simulink model "NREL5MW_FBSWE_SLOW3DOF_IPC"  (R2021b)
settings: Solver=ode4  StartTime=0.0  StopTime=Parameter.Time.TMax  FixedStep=Parameter.Time.dt  RelTol=1e-3  EnableMultiTasking=on
values from neighbouring files (symbols this model uses):
  Parameter = NREL5MWDefaultParameter_FBSWE_IPC(Parameter)    [Exercise09_IndividualPitchControllerTest.m]
undefined symbols (not defined in the file or in its folder): x2_max, x2_min, x2_t0
libraries: simulink x4
(part 1 of 2)
settings Model: Creator=Phoenix_Shao  LastModifiedBy=david
settings SolverCC: AlgebraicLoopSolver=TrustRegion
settings DataIOCC: MaxDataPoints=1000000  SaveFormat=Array  DSMLogging=off  ReturnWorkspaceOutputs=off
settings OptimizationCC: ExpressionDepthLimit=2147483647  InitFltsAndDblsToZero=on  EfficientMapNaN2IntZero=off  LifeSpan=inf
settings DebuggingCC: SaveWithParameterizedLinksMsg=none  UnderspecifiedInitializationDetection=Classic  MergeDetectMultiDrivingBlocksExec=none  SignalResolutionControl=TryResolveAllWithWarning  SolverPrmCheckMsg=warning  MultiTaskDSMMsg=warning  MultiTaskCondExecSysMsg=none  FcnCallInpInsideContextMsg=warning  AllowSymbolicDim=off  StateNameClashWarn=warning  SFUnexpectedBacktrackingDiag=warning  SFNoUnconditionalDefaultTransitionDiag=warning  SFExecutionAtInitializationDiag=none  SFMachineParentedDataDiag=warning  ArithmeticOperatorsInVariantConditions=warning
settings HardwareCC: ProdBitPerPointer=32  ProdBitPerSizeT=32  ProdBitPerPtrDiffT=32  ProdLargestAtomicFloat=None  ProdIntDivRoundTo=Undefined  ProdEndianess=Unspecified  ProdWordSize=32  ProdHWDeviceType=32-bit Generic  TargetBitPerPointer=64  TargetBitPerSizeT=64  TargetBitPerPtrDiffT=64  TargetLongLongMode=on  TargetIntDivRoundTo=Zero  TargetEndianess=LittleEndian  TargetWordSize=64  TargetHWDeviceType=MATLAB Host  ProdEqTarget=off
settings ModelReferenceCC: PropagateSignalLabelsOutOfModel=off
settings SFSimCC: SimUseLocalCustomCode=off  SimParseCustomCode=off  CustomCodeUndefinedFunction=UseInterfaceOnly
settings RTWCC: SystemTargetFile=accel.tlc  TemplateMakefile=accel_default_tmf  RTWVerbose=off  RTWUseLocalCustomCode=off
settings CodeAppCC: MaxIdLength=128  StateflowObjectComments=on
settings STFCustomTargetCC: MATLABClassNameForMDSCustomization=Simulink.SoftwareTarget.TargetSpecificTriggerConfigurationBase  SystemTargetFile=accel.tlc
settings ConfigComp: CovMetricSettings=dw  CovSaveCumulativeToWorkspaceVar=on  CovSaveSingleToWorkspaceVar=on  CovExternalEMLEnable=off

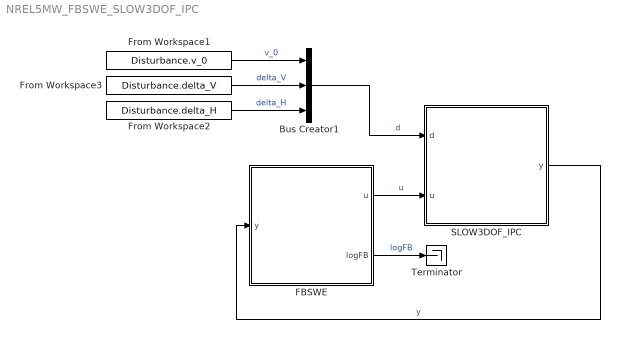
== system NREL5MW_FBSWE_SLOW3DOF_IPC ==
  Bus Creator1 : BusCreator  Inputs=3
  FBSWE : Subsystem
  From Workspace1 : FromWorkspace  VariableName=Disturbance.v_0
  From Workspace2 : FromWorkspace  VariableName=Disturbance.delta_H
  From Workspace3 : FromWorkspace  VariableName=Disturbance.delta_V
  SLOW3DOF_IPC : Subsystem
  Terminator : Terminator
  wires:
  SLOW3DOF_IPC/1(y) -> FBSWE/1(y)  "y"
  FBSWE/2(logFB) -> Terminator/1  "logFB"
  From Workspace1/1 -> Bus Creator1/1  "v_0"
  From Workspace3/1 -> Bus Creator1/2  "delta_V"
  From Workspace2/1 -> Bus Creator1/3  "delta_H"
  FBSWE/1(u) -> SLOW3DOF_IPC/2(u)  "u"
  Bus Creator1/1 -> SLOW3DOF_IPC/1(d)  "d"

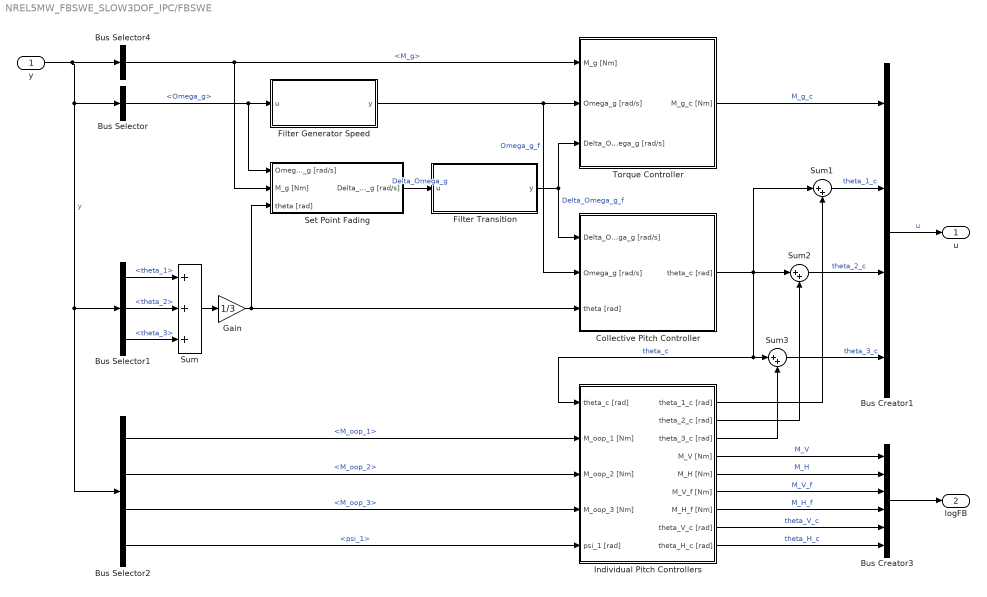
== system NREL5MW_FBSWE_SLOW3DOF_IPC/FBSWE ==
  y : Inport
  Bus Creator1 : BusCreator  Inputs=4
  Bus Creator3 : BusCreator  Inputs=6
  Bus Selector : BusSelector  OutputSignals=Omega_g
  Bus Selector1 : BusSelector  OutputSignals=theta_1,theta_2,theta_3
  Bus Selector2 : BusSelector  OutputSignals=M_oop_1,M_oop_2,M_oop_3,psi_1
  Bus Selector4 : BusSelector  OutputSignals=M_g
  Collective Pitch Controller : Subsystem
  Filter Generator Speed : Subsystem
  Filter Transition : Subsystem
  Gain : Gain  Gain=1/3
  Individual Pitch Controllers : Subsystem
  Set Point Fading : Subsystem
  Sum : Sum  Inputs=+++
  Sum1 : Sum  Inputs=|++
  Sum2 : Sum  Inputs=|++
  Sum3 : Sum  Inputs=|++
  Torque Controller : Subsystem
  u : Outport  VectorParamsAs1DForOutWhenUnconnected=off
  logFB : Outport  Port=2  VectorParamsAs1DForOutWhenUnconnected=off
  wires:
  Bus Selector/1 -> Set Point Fading/1(Omega_g [rad/s]), Filter Generator Speed/1(u)  "<Omega_g>"
  y/1 -> Bus Selector/1, Bus Selector2/1, Bus Selector1/1, Bus Selector4/1  "y"
  Torque Controller/1(M_g_c [Nm]) -> Bus Creator1/1  "M_g_c"
  Bus Creator1/1 -> u/1  "u"
  Filter Generator Speed/1(y) -> Collective Pitch Controller/2(Omega_g [rad/s]), Torque Controller/2(Omega_g [rad/s])  "Omega_g_f"
  Bus Selector4/1 -> Set Point Fading/2(M_g [Nm]), Torque Controller/1(M_g [Nm])  "<M_g>"
  Set Point Fading/1(Delta_Omega_g [rad/s]) -> Filter Transition/1(u)  "Delta_Omega_g"
  Filter Transition/1(y) -> Collective Pitch Controller/1(Delta_Omega_g [rad/s]), Torque Controller/3(Delta_Omega_g [rad/s])  "Delta_Omega_g_f"
  Bus Selector1/1 -> Sum/1  "<theta_1>"
  Bus Selector1/2 -> Sum/2  "<theta_2>"
  Bus Selector1/3 -> Sum/3  "<theta_3>"
  Sum/1 -> Gain/1
  Gain/1 -> Set Point Fading/3(theta [rad]), Collective Pitch Controller/3(theta [rad])
  Sum1/1 -> Bus Creator1/2  "theta_1_c"
  Sum2/1 -> Bus Creator1/3  "theta_2_c"
  Sum3/1 -> Bus Creator1/4  "theta_3_c"
  Collective Pitch Controller/1(theta_c [rad]) -> Sum1/1, Individual Pitch Controllers/1(theta_c [rad]), Sum3/1, Sum2/1  "theta_c"
  Bus Selector2/1 -> Individual Pitch Controllers/2(M_oop_1 [Nm])  "<M_oop_1>"
  Bus Selector2/2 -> Individual Pitch Controllers/3(M_oop_2 [Nm])  "<M_oop_2>"
  Bus Selector2/3 -> Individual Pitch Controllers/4(M_oop_3 [Nm])  "<M_oop_3>"
  Bus Selector2/4 -> Individual Pitch Controllers/5(psi_1 [rad])  "<psi_1>"
  Individual Pitch Controllers/1(theta_1_c [rad]) -> Sum1/2
  Individual Pitch Controllers/2(theta_2_c [rad]) -> Sum2/2
  Individual Pitch Controllers/3(theta_3_c [rad]) -> Sum3/2
  Bus Creator3/1 -> logFB/1
  Individual Pitch Controllers/4(M_V [Nm]) -> Bus Creator3/1  "M_V"
  Individual Pitch Controllers/5(M_H [Nm]) -> Bus Creator3/2  "M_H"
  Individual Pitch Controllers/9(theta_H_c [rad]) -> Bus Creator3/6  "theta_H_c"
  Individual Pitch Controllers/8(theta_V_c [rad]) -> Bus Creator3/5  "theta_V_c"
  Individual Pitch Controllers/6(M_V_f [Nm]) -> Bus Creator3/3  "M_V_f"
  Individual Pitch Controllers/7(M_H_f [Nm]) -> Bus Creator3/4  "M_H_f"

== system NREL5MW_FBSWE_SLOW3DOF_IPC/SLOW3DOF_IPC ==
  d : Inport
  u : Inport  Port=2
  Bus Creator1 : BusCreator  Inputs=10
  Bus Selector : BusSelector  OutputSignals=theta_1_c,theta_2_c,theta_3_c
  Bus Selector1 : BusSelector  OutputSignals=M_g_c
  Bus Selector3 : BusSelector  OutputSignals=v_0,delta_V,delta_H
  aerodynamics : Subsystem
  drive-train dynamics : Subsystem
  generator : Subsystem
  pitch actuators : Subsystem
  rotational sampling wind : Subsystem
  tower fore-aft dynamics : Subsystem
  y : Outport  VectorParamsAs1DForOutWhenUnconnected=off
  wires:
  u/1 -> Bus Selector1/1, Bus Selector/1
  aerodynamics/5(F_a [N]) -> tower fore-aft dynamics/1(F_a [N])  "F_a"
  aerodynamics/1(M_a [Nm]) -> drive-train dynamics/2(M_a [Nm])  "M_a"
  drive-train dynamics/2(Omega [rad/s]) -> aerodynamics/1(Omega [rad/s])  "Omega"
  drive-train dynamics/3(Omega_g [rad/s]) -> generator/1(Omega_g [rad/s]), Bus Creator1/3  "Omega_g"
  pitch actuators/1(theta_1 [rad]) -> Bus Creator1/8, aerodynamics/5(theta_1 [rad])  "theta_1"
  Bus Selector1/1 -> generator/2(M_g_c [Nm])  "<M_g_c>"
  d/1 -> Bus Selector3/1
  Bus Selector3/3 -> rotational sampling wind/3(delta_H [1/s])  "<delta_H>"
  Bus Selector3/1 -> rotational sampling wind/1(v_0 [m/s])  "<v_0>"
  Bus Selector3/2 -> rotational sampling wind/2(delta_V [1/s])  "<delta_V>"
  generator/1(M_g [Nm]) -> drive-train dynamics/1(M_g [Nm]), Bus Creator1/1  "M_g"
  rotational sampling wind/3(v_3 [m/s]) -> aerodynamics/4(v_3 [m/s])  "v_3"
  rotational sampling wind/2(v_2 [m/s]) -> aerodynamics/3(v_2 [m/s])  "v_2"
  rotational sampling wind/1(v_1 [m/s]) -> aerodynamics/2(v_1 [m/s])  "v_1"
  pitch actuators/2(theta_2 [rad]) -> Bus Creator1/9, aerodynamics/6(theta_2 [rad])  "theta_2"
  pitch actuators/3(theta_3 [rad]) -> Bus Creator1/10, aerodynamics/7(theta_3 [rad])  "theta_3"
  tower fore-aft dynamics/2(x_T_dot [m/s]) -> aerodynamics/8(x_T_dot [m/s])  "x_T_dot"
  aerodynamics/2(M_oop_1 [Nm]) -> Bus Creator1/4  "M_oop_1"
  aerodynamics/3(M_oop_2 [Nm]) -> Bus Creator1/5  "M_oop_2"
  aerodynamics/4(M_oop_3 [Nm]) -> Bus Creator1/6  "M_oop_3"
  tower fore-aft dynamics/1(x_T_dotdot [m/s^2]) -> Bus Creator1/7  "x_T_dotdot"
  Bus Selector/1 -> pitch actuators/1(theta_1_c [rad])  "<theta_1_c>"
  Bus Selector/2 -> pitch actuators/2(theta_2_c [rad])  "<theta_2_c>"
  Bus Selector/3 -> pitch actuators/3(theta_3_c [rad])  "<theta_3_c>"
  Bus Creator1/1 -> y/1
  drive-train dynamics/1(psi_1 [rad]) -> rotational sampling wind/4(psi_1 [rad/s]), Bus Creator1/2  "psi_1"

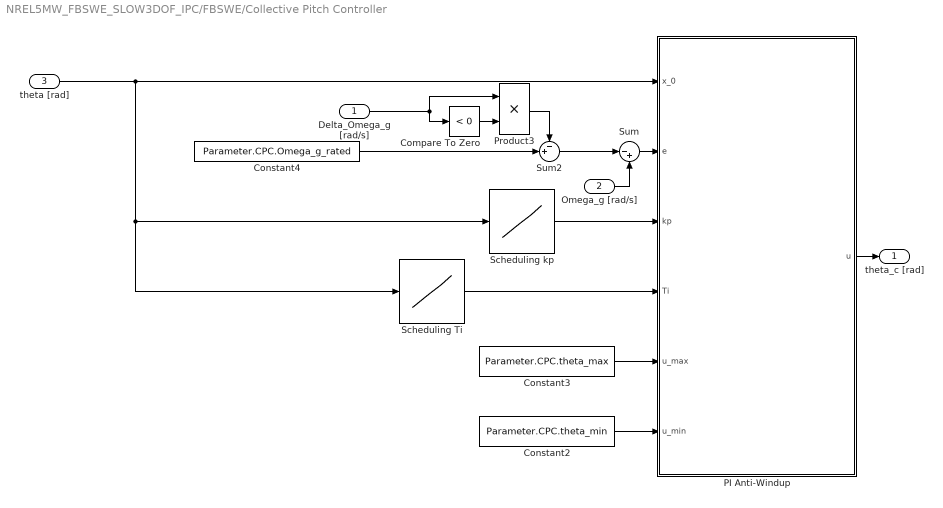
== system NREL5MW_FBSWE_SLOW3DOF_IPC/FBSWE/Collective Pitch Controller ==
  Delta_Omega_g [rad/s] : Inport
  Omega_g [rad/s] : Inport  Port=2
  theta [rad] : Inport  Port=3
  Compare To Zero : simulink/Logic and Bit Operations/Compare To Zero  relop=<  OutDataTypeStr=boolean
  Constant2 : Constant  Value=Parameter.CPC.theta_min
  Constant3 : Constant  Value=Parameter.CPC.theta_max
  Constant4 : Constant  Value=Parameter.CPC.Omega_g_rated
  PI Anti-Windup : Subsystem
  Product3 : Product
  Scheduling Ti : Lookup_n-D  NumberOfTableDimensions=1  BreakpointsForDimension1=Parameter.CPC.GS.theta  IndexSearchMethod=Linear search  Table=Parameter.CPC.GS.Ti  ExtrapMethod=Clip  UseLastTableValue=on  InternalRulePriority=Speed  RndMeth=Simplest  InputSameDT=on
  Scheduling kp : Lookup_n-D  NumberOfTableDimensions=1  BreakpointsForDimension1=Parameter.CPC.GS.theta  IndexSearchMethod=Linear search  Table=Parameter.CPC.GS.kp  ExtrapMethod=Clip  UseLastTableValue=on  InternalRulePriority=Speed  RndMeth=Simplest  InputSameDT=on
  Sum : Sum  Inputs=|-+
  Sum2 : Sum  Inputs=-+|
  theta_c [rad] : Outport  VectorParamsAs1DForOutWhenUnconnected=off
  wires:
  Scheduling Ti/1 -> PI Anti-Windup/4(Ti)
  Scheduling kp/1 -> PI Anti-Windup/3(kp)
  theta [rad]/1 -> PI Anti-Windup/1(x_0), Scheduling kp/1, Scheduling Ti/1
  Omega_g [rad/s]/1 -> Sum/2
  Sum/1 -> PI Anti-Windup/2(e)
  PI Anti-Windup/1(u) -> theta_c [rad]/1
  Constant2/1 -> PI Anti-Windup/6(u_min)
  Constant3/1 -> PI Anti-Windup/5(u_max)
  Delta_Omega_g [rad/s]/1 -> Product3/1, Compare To Zero/1
  Compare To Zero/1 -> Product3/2
  Product3/1 -> Sum2/1
  Constant4/1 -> Sum2/2
  Sum2/1 -> Sum/1

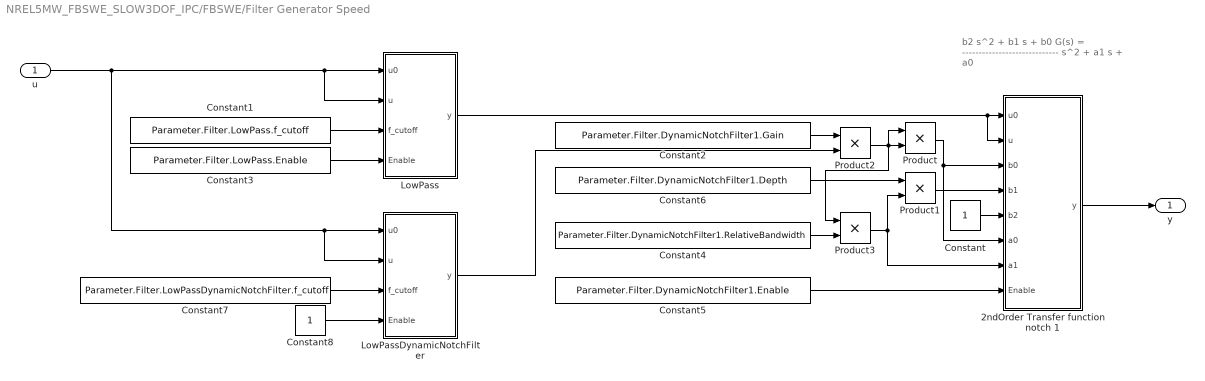
== system NREL5MW_FBSWE_SLOW3DOF_IPC/FBSWE/Filter Generator Speed ==
  note: b2 s^2 + b1 s + b0
      | G(s) = -----------------------------
      | s^2 + a1 s + a0
  u : Inport
  2ndOrder Transfer function notch 1 : Subsystem
  Constant : Constant
  Constant1 : Constant  Value=Parameter.Filter.LowPass.f_cutoff
  Constant2 : Constant  Value=Parameter.Filter.DynamicNotchFilter1.Gain
  Constant3 : Constant  Value=Parameter.Filter.LowPass.Enable
  Constant4 : Constant  Value=Parameter.Filter.DynamicNotchFilter1.RelativeBandwidth
  Constant5 : Constant  Value=Parameter.Filter.DynamicNotchFilter1.Enable
  Constant6 : Constant  Value=Parameter.Filter.DynamicNotchFilter1.Depth
  Constant7 : Constant  Value=Parameter.Filter.LowPassDynamicNotchFilter.f_cutoff
  Constant8 : Constant
  LowPass : Subsystem
  LowPassDynamicNotchFilter : Subsystem
  Product{,1..3} (4 alike) : Product  RndMeth=Zero
  y : Outport  VectorParamsAs1DForOutWhenUnconnected=off
  wires:
  Constant3/1 -> LowPass/4(Enable)
  Constant1/1 -> LowPass/3(f_cutoff)
  LowPassDynamicNotchFilter/1(y) -> Product2/2
  Product2/1 -> Product3/1, Product/1, Product/2
  Constant2/1 -> Product2/1
  Constant/1 -> 2ndOrder Transfer function notch 1/5(b2)
  Product1/1 -> 2ndOrder Transfer function notch 1/4(b1)
  2ndOrder Transfer function notch 1/1(y) -> y/1
  Constant4/1 -> Product3/2
  Constant6/1 -> Product1/1
  Product/1 -> 2ndOrder Transfer function notch 1/3(b0), 2ndOrder Transfer function notch 1/6(a0)
  LowPass/1(y) -> 2ndOrder Transfer function notch 1/2(u), 2ndOrder Transfer function notch 1/1(u0)
  Constant5/1 -> 2ndOrder Transfer function notch 1/8(Enable)
  Constant7/1 -> LowPassDynamicNotchFilter/3(f_cutoff)
  Constant8/1 -> LowPassDynamicNotchFilter/4(Enable)
  u/1 -> LowPassDynamicNotchFilter/1(u0), LowPassDynamicNotchFilter/2(u), LowPass/2(u), LowPass/1(u0)
  Product3/1 -> 2ndOrder Transfer function notch 1/7(a1), Product1/2

== system NREL5MW_FBSWE_SLOW3DOF_IPC/FBSWE/Filter Transition ==
  u : Inport
  Constant1 : Constant  Value=Parameter.Filter.LowPass2.f_cutoff
  LowPassOrder1 : Subsystem
  y : Outport  VectorParamsAs1DForOutWhenUnconnected=off
  wires:
  LowPassOrder1/1(y) -> y/1
  Constant1/1 -> LowPassOrder1/3(f_cutoff)
  u/1 -> LowPassOrder1/1(u0), LowPassOrder1/2(u)

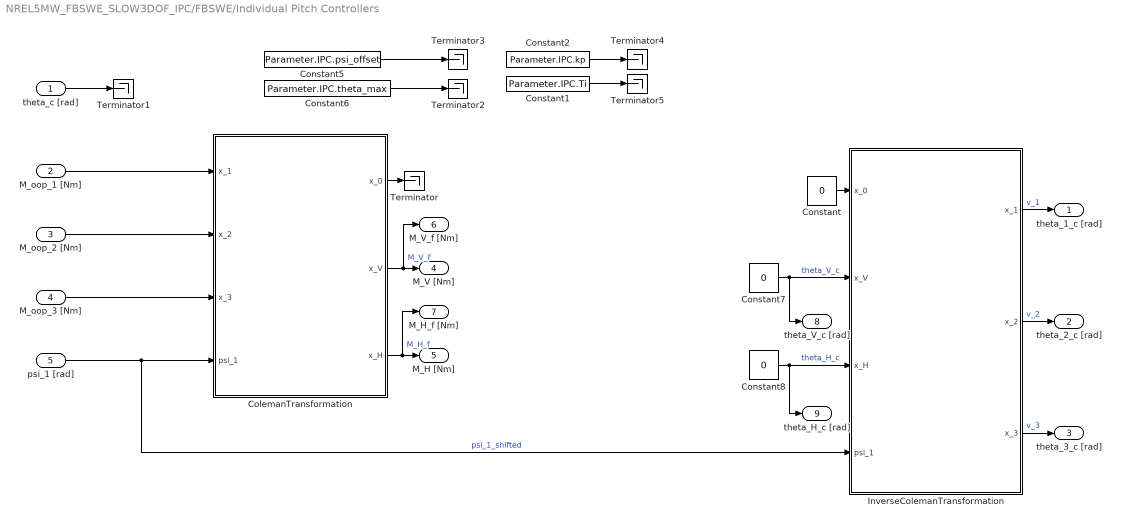
== system NREL5MW_FBSWE_SLOW3DOF_IPC/FBSWE/Individual Pitch Controllers ==
  theta_c [rad] : Inport
  M_oop_1 [Nm] : Inport  Port=2
  M_oop_2 [Nm] : Inport  Port=3
  M_oop_3 [Nm] : Inport  Port=4
  psi_1 [rad] : Inport  Port=5
  ColemanTransformation : MATLAB Function  TreatAsAtomicUnit=on
  Constant : Constant  Value=0
  Constant1 : Constant  Value=Parameter.IPC.Ti
  Constant2 : Constant  Value=Parameter.IPC.kp
  Constant5 : Constant  Value=Parameter.IPC.psi_offset
  Constant6 : Constant  Value=Parameter.IPC.theta_max
  Constant7 : Constant  Value=0
  Constant8 : Constant  Value=0
  InverseColemanTransformation : MATLAB Function  TreatAsAtomicUnit=on
  Terminator{,1..5} (6 alike) : Terminator
  theta_1_c [rad] : Outport  VectorParamsAs1DForOutWhenUnconnected=off
  theta_2_c [rad] : Outport  Port=2  VectorParamsAs1DForOutWhenUnconnected=off
  theta_3_c [rad] : Outport  Port=3  VectorParamsAs1DForOutWhenUnconnected=off
  M_V [Nm] : Outport  Port=4  VectorParamsAs1DForOutWhenUnconnected=off
  M_H [Nm] : Outport  Port=5  VectorParamsAs1DForOutWhenUnconnected=off
  M_V_f [Nm] : Outport  Port=6  VectorParamsAs1DForOutWhenUnconnected=off
  M_H_f [Nm] : Outport  Port=7  VectorParamsAs1DForOutWhenUnconnected=off
  theta_V_c [rad] : Outport  Port=8  VectorParamsAs1DForOutWhenUnconnected=off
  theta_H_c [rad] : Outport  Port=9  VectorParamsAs1DForOutWhenUnconnected=off
  wires:
  ColemanTransformation/1(x_0) -> Terminator/1
  Constant7/1 -> theta_V_c [rad]/1, InverseColemanTransformation/2(x_V)  "theta_V_c"
  Constant8/1 -> theta_H_c [rad]/1, InverseColemanTransformation/3(x_H)  "theta_H_c"
  InverseColemanTransformation/1(x_1) -> theta_1_c [rad]/1  "v_1"
  InverseColemanTransformation/2(x_2) -> theta_2_c [rad]/1  "v_2"
  InverseColemanTransformation/3(x_3) -> theta_3_c [rad]/1  "v_3"
  Constant/1 -> InverseColemanTransformation/1(x_0)
  psi_1 [rad]/1 -> InverseColemanTransformation/4(psi_1), ColemanTransformation/4(psi_1)  "psi_1_shifted"
  M_oop_1 [Nm]/1 -> ColemanTransformation/1(x_1)
  M_oop_2 [Nm]/1 -> ColemanTransformation/2(x_2)
  M_oop_3 [Nm]/1 -> ColemanTransformation/3(x_3)
  ColemanTransformation/2(x_V) -> M_V_f [Nm]/1, M_V [Nm]/1  "M_V_f"
  ColemanTransformation/3(x_H) -> M_H_f [Nm]/1, M_H [Nm]/1  "M_H_f"
  Constant6/1 -> Terminator2/1
  theta_c [rad]/1 -> Terminator1/1
  Constant5/1 -> Terminator3/1
  Constant2/1 -> Terminator4/1
  Constant1/1 -> Terminator5/1

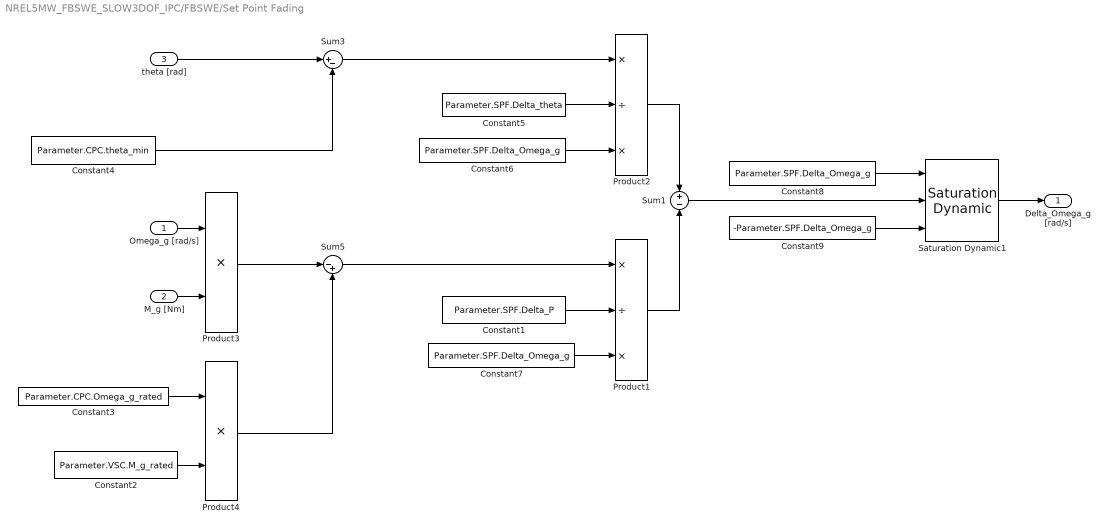
== system NREL5MW_FBSWE_SLOW3DOF_IPC/FBSWE/Set Point Fading ==
  Omega_g [rad/s] : Inport
  M_g [Nm] : Inport  Port=2
  theta [rad] : Inport  Port=3
  Constant1 : Constant  Value=Parameter.SPF.Delta_P
  Constant2 : Constant  Value=Parameter.VSC.M_g_rated
  Constant3 : Constant  Value=Parameter.CPC.Omega_g_rated
  Constant4 : Constant  Value=Parameter.CPC.theta_min
  Constant5 : Constant  Value=Parameter.SPF.Delta_theta
  Constant6 : Constant  Value=Parameter.SPF.Delta_Omega_g
  Constant7 : Constant  Value=Parameter.SPF.Delta_Omega_g
  Constant8 : Constant  Value=Parameter.SPF.Delta_Omega_g
  Constant9 : Constant  Value=-Parameter.SPF.Delta_Omega_g
  Product1 : Product  Inputs=*/*  RndMeth=Zero
  Product2 : Product  Inputs=*/*  RndMeth=Zero
  Product3 : Product  RndMeth=Zero
  Product4 : Product  RndMeth=Zero
  Saturation Dynamic1 : simulink/Discontinuities/Saturation Dynamic  OutMin=[]  OutMax=[]  OutDataTypeStr=Inherit: Same as second input  OutDataType=fixdt(1, 16)  OutScaling=2^-10  DoSatur=off
  Sum1 : Sum  Inputs=+|-
  Sum3 : Sum  Inputs=|+-
  Sum5 : Sum  Inputs=|-+
  Delta_Omega_g [rad/s] : Outport  VectorParamsAs1DForOutWhenUnconnected=off
  wires:
  theta [rad]/1 -> Sum3/1
  Sum3/1 -> Product2/1
  Product2/1 -> Sum1/1
  Constant5/1 -> Product2/2
  Constant4/1 -> Sum3/2
  Sum5/1 -> Product1/1
  Product1/1 -> Sum1/2
  M_g [Nm]/1 -> Product3/2
  Omega_g [rad/s]/1 -> Product3/1
  Product3/1 -> Sum5/1
  Constant2/1 -> Product4/2
  Constant3/1 -> Product4/1
  Product4/1 -> Sum5/2
  Constant6/1 -> Product2/3
  Constant1/1 -> Product1/2
  Constant7/1 -> Product1/3
  Saturation Dynamic1/1 -> Delta_Omega_g [rad/s]/1
  Sum1/1 -> Saturation Dynamic1/2
  Constant8/1 -> Saturation Dynamic1/1
  Constant9/1 -> Saturation Dynamic1/3

== system NREL5MW_FBSWE_SLOW3DOF_IPC/FBSWE/Torque Controller ==
  M_g [Nm] : Inport
  Omega_g [rad/s] : Inport  Port=2
  Delta_Omega_g [rad/s] : Inport  Port=3
  Constant : Constant  Value=Parameter.VSC.kp
  Constant1 : Constant  Value=Parameter.VSC.Ti
  LimitsAndReferenceValueTC : Subsystem
  PI Anti-Windup : Subsystem
  Sum : Sum  Inputs=|+-
  M_g_c [Nm] : Outport  VectorParamsAs1DForOutWhenUnconnected=off
  wires:
  LimitsAndReferenceValueTC/1(Omega_g_ref [rad/s]) -> Sum/2
  M_g [Nm]/1 -> PI Anti-Windup/1(x_0)
  Sum/1 -> PI Anti-Windup/2(e)
  Constant/1 -> PI Anti-Windup/3(kp)
  Constant1/1 -> PI Anti-Windup/4(Ti)
  Omega_g [rad/s]/1 -> LimitsAndReferenceValueTC/1(Omega_g [rad/s]), Sum/1
  LimitsAndReferenceValueTC/2(M_g_ub [Nm]) -> PI Anti-Windup/5(u_max)  "M_g_ub"
  LimitsAndReferenceValueTC/3(M_g_lb [Nm]) -> PI Anti-Windup/6(u_min)  "M_g_lb"
  PI Anti-Windup/1(u) -> M_g_c [Nm]/1
  Delta_Omega_g [rad/s]/1 -> LimitsAndReferenceValueTC/2(Delta_Omega_g [rad/s])

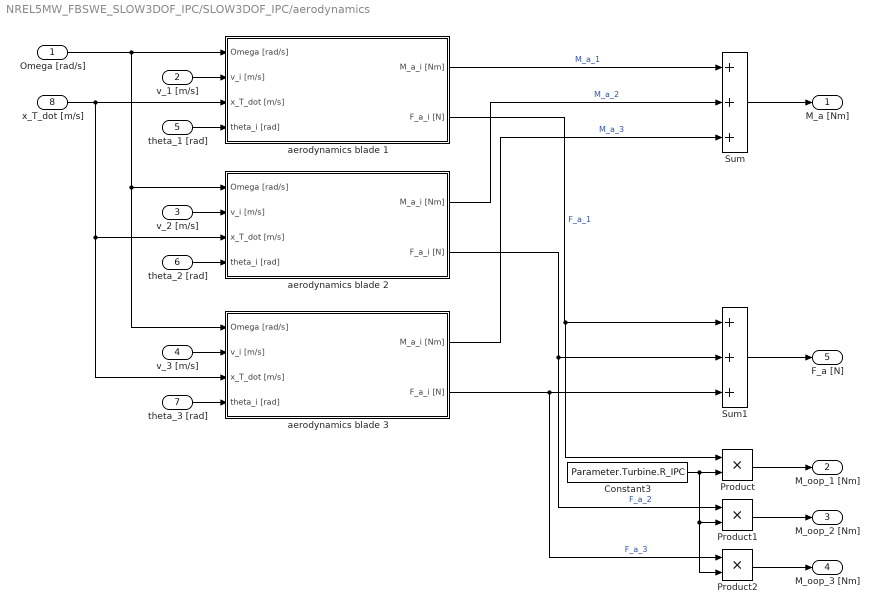
== system NREL5MW_FBSWE_SLOW3DOF_IPC/SLOW3DOF_IPC/aerodynamics ==
  Omega [rad/s] : Inport
  v_1 [m/s] : Inport  Port=2
  v_2 [m/s] : Inport  Port=3
  v_3 [m/s] : Inport  Port=4
  theta_1 [rad] : Inport  Port=5
  theta_2 [rad] : Inport  Port=6
  theta_3 [rad] : Inport  Port=7
  x_T_dot [m/s] : Inport  Port=8
  Constant3 : Constant  Value=Parameter.Turbine.R_IPC
  Product : Product
  Product1 : Product
  Product2 : Product
  Sum : Sum  Inputs=+++
  Sum1 : Sum  Inputs=+++
  aerodynamics blade 1 : Subsystem
  aerodynamics blade 2 : Subsystem
  aerodynamics blade 3 : Subsystem
  M_a [Nm] : Outport  VectorParamsAs1DForOutWhenUnconnected=off
  M_oop_1 [Nm] : Outport  Port=2  VectorParamsAs1DForOutWhenUnconnected=off
  M_oop_2 [Nm] : Outport  Port=3  VectorParamsAs1DForOutWhenUnconnected=off
  M_oop_3 [Nm] : Outport  Port=4  VectorParamsAs1DForOutWhenUnconnected=off
  F_a [N] : Outport  Port=5  VectorParamsAs1DForOutWhenUnconnected=off
  wires:
  Sum/1 -> M_a [Nm]/1
  Sum1/1 -> F_a [N]/1
  x_T_dot [m/s]/1 -> aerodynamics blade 3/3(x_T_dot [m/s]), aerodynamics blade 2/3(x_T_dot [m/s]), aerodynamics blade 1/3(x_T_dot [m/s])
  v_1 [m/s]/1 -> aerodynamics blade 1/2(v_i [m/s])
  Omega [rad/s]/1 -> aerodynamics blade 3/1(Omega [rad/s]), aerodynamics blade 2/1(Omega [rad/s]), aerodynamics blade 1/1(Omega [rad/s])
  theta_1 [rad]/1 -> aerodynamics blade 1/4(theta_i [rad])
  v_2 [m/s]/1 -> aerodynamics blade 2/2(v_i [m/s])
  v_3 [m/s]/1 -> aerodynamics blade 3/2(v_i [m/s])
  theta_3 [rad]/1 -> aerodynamics blade 3/4(theta_i [rad])
  theta_2 [rad]/1 -> aerodynamics blade 2/4(theta_i [rad])
  aerodynamics blade 1/1(M_a_i [Nm]) -> Sum/1  "M_a_1"
  aerodynamics blade 2/1(M_a_i [Nm]) -> Sum/2  "M_a_2"
  aerodynamics blade 3/1(M_a_i [Nm]) -> Sum/3  "M_a_3"
  aerodynamics blade 3/2(F_a_i [N]) -> Product2/1, Sum1/3  "F_a_3"
  aerodynamics blade 2/2(F_a_i [N]) -> Product1/1, Sum1/2  "F_a_2"
  aerodynamics blade 1/2(F_a_i [N]) -> Product/1, Sum1/1  "F_a_1"
  Product/1 -> M_oop_1 [Nm]/1
  Constant3/1 -> Product2/2, Product1/2, Product/2
  Product2/1 -> M_oop_3 [Nm]/1
  Product1/1 -> M_oop_2 [Nm]/1

== system NREL5MW_FBSWE_SLOW3DOF_IPC/SLOW3DOF_IPC/drive-train dynamics ==
  M_g [Nm] : Inport
  M_a [Nm] : Inport  Port=2
  Add4 : Sum  Inputs=-+
  Gain12 : Gain  Gain=Parameter.Turbine.r_GB  SaturateOnIntegerOverflow=on  OutDataTypeStr=Inherit: Same as input  ParamDataTypeStr=Inherit: Same as input
  Gain2 : Gain  Gain=Parameter.Turbine.r_GB  SaturateOnIntegerOverflow=on  OutDataTypeStr=Inherit: Same as input  ParamDataTypeStr=Inherit: Same as input
  Gain8 : Gain  Gain=1/Parameter.Turbine.J  SaturateOnIntegerOverflow=on  OutDataTypeStr=Inherit: Same as input  ParamDataTypeStr=Inherit: Same as input
  Integrator : Integrator
  Integrator4 : Integrator  InitialCondition=Parameter.IC.Omega
  psi_1 [rad] : Outport  VectorParamsAs1DForOutWhenUnconnected=off
  Omega [rad/s] : Outport  Port=2  VectorParamsAs1DForOutWhenUnconnected=off
  Omega_g [rad/s] : Outport  Port=3  VectorParamsAs1DForOutWhenUnconnected=off
  wires:
  Integrator/1 -> psi_1 [rad]/1
  Gain2/1 -> Add4/1
  Add4/1 -> Gain8/1
  M_g [Nm]/1 -> Gain2/1  "M_g"
  Gain12/1 -> Omega_g [rad/s]/1  "Omega_g [rad/s]"
  Gain8/1 -> Integrator4/1
  M_a [Nm]/1 -> Add4/2  "M_a"
  Integrator4/1 -> Integrator/1, Omega [rad/s]/1, Gain12/1  "Omega"

== system NREL5MW_FBSWE_SLOW3DOF_IPC/SLOW3DOF_IPC/generator ==
  Omega_g [rad/s] : Inport
  M_g_c [Nm] : Inport  Port=2
  Constant3 : Constant  Value=Parameter.Generator.eta_el
  Product1 : Product  Inputs=***  RndMeth=Zero
  Simple Torque Actuator : Memory  InitialCondition=Parameter.IC.M_g
  Terminator4 : Terminator
  M_g [Nm] : Outport  VectorParamsAs1DForOutWhenUnconnected=off
  wires:
  Constant3/1 -> Product1/3
  M_g_c [Nm]/1 -> Simple Torque Actuator/1
  Omega_g [rad/s]/1 -> Product1/2
  Product1/1 -> Terminator4/1  "P_el"
  Simple Torque Actuator/1 -> M_g [Nm]/1, Product1/1  "M_g"

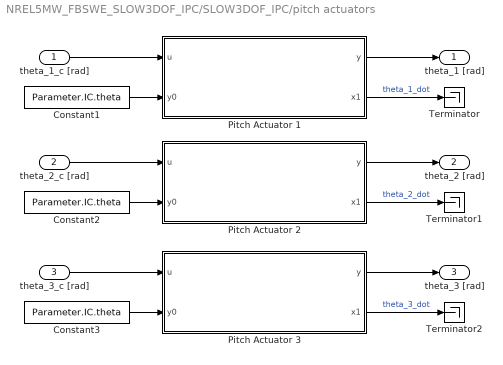
== system NREL5MW_FBSWE_SLOW3DOF_IPC/SLOW3DOF_IPC/pitch actuators ==
  theta_1_c [rad] : Inport
  theta_2_c [rad] : Inport  Port=2
  theta_3_c [rad] : Inport  Port=3
  Constant1 : Constant  Value=Parameter.IC.theta
  Constant2 : Constant  Value=Parameter.IC.theta
  Constant3 : Constant  Value=Parameter.IC.theta
  Pitch Actuator 1 : Subsystem  mask{omega=Parameter.PitchActuator.omega, xi=Parameter.PitchActuator.xi, x1_max=Parameter.PitchActuator.theta_dot_max, x1_min=-Parameter.PitchActuator.theta_dot_max}
      mask prompts: omega "undamped natural frequency [rad/s]"; xi "damping factor [-]"; x1_max "Upper bound x1"; x1_min "Lower bound x1"
      mask Display:
      | disp(['omega = ',num2str(omega),'\n'...
      |     ,'xi = ',num2str(xi)])
      | port_label('output',1,'y')
      | port_label('output',2,'x1')
      | port_label('input',2,'y0')
      | port_label('input',1,'u')
  Pitch Actuator 2 : Subsystem  mask{omega=Parameter.PitchActuator.omega, xi=Parameter.PitchActuator.xi, x1_max=Parameter.PitchActuator.theta_dot_max, x1_min=-Parameter.PitchActuator.theta_dot_max}
      mask prompts: omega "undamped natural frequency [rad/s]"; xi "damping factor [-]"; x1_max "Upper bound x1"; x1_min "Lower bound x1"
      mask Display:
      | disp(['omega = ',num2str(omega),'\n'...
      |     ,'xi = ',num2str(xi)])
      | port_label('output',1,'y')
      | port_label('output',2,'x1')
      | port_label('input',2,'y0')
      | port_label('input',1,'u')
  Pitch Actuator 3 : Subsystem  mask{omega=Parameter.PitchActuator.omega, xi=Parameter.PitchActuator.xi, x1_max=Parameter.PitchActuator.theta_dot_max, x1_min=-Parameter.PitchActuator.theta_dot_max}
      mask prompts: omega "undamped natural frequency [rad/s]"; xi "damping factor [-]"; x1_max "Upper bound x1"; x1_min "Lower bound x1"
      mask Display:
      | disp(['omega = ',num2str(omega),'\n'...
      |     ,'xi = ',num2str(xi)])
      | port_label('output',1,'y')
      | port_label('output',2,'x1')
      | port_label('input',2,'y0')
      | port_label('input',1,'u')
  Terminator : Terminator
  Terminator1 : Terminator
  Terminator2 : Terminator
  theta_1 [rad] : Outport  VectorParamsAs1DForOutWhenUnconnected=off
  theta_2 [rad] : Outport  Port=2  VectorParamsAs1DForOutWhenUnconnected=off
  theta_3 [rad] : Outport  Port=3  VectorParamsAs1DForOutWhenUnconnected=off
  wires:
  theta_1_c [rad]/1 -> Pitch Actuator 1/1(u)
  Constant1/1 -> Pitch Actuator 1/2(y0)
  Pitch Actuator 1/2(x1) -> Terminator/1  "theta_1_dot"
  Pitch Actuator 2/2(x1) -> Terminator1/1  "theta_2_dot"
  Constant2/1 -> Pitch Actuator 2/2(y0)
  theta_2_c [rad]/1 -> Pitch Actuator 2/1(u)
  theta_3_c [rad]/1 -> Pitch Actuator 3/1(u)
  Constant3/1 -> Pitch Actuator 3/2(y0)
  Pitch Actuator 3/2(x1) -> Terminator2/1  "theta_3_dot"
  Pitch Actuator 1/1(y) -> theta_1 [rad]/1
  Pitch Actuator 3/1(y) -> theta_3 [rad]/1
  Pitch Actuator 2/1(y) -> theta_2 [rad]/1

== system NREL5MW_FBSWE_SLOW3DOF_IPC/SLOW3DOF_IPC/rotational sampling wind ==
  v_0 [m/s] : Inport
  delta_V [1/s] : Inport  Port=2
  delta_H [1/s] : Inport  Port=3
  psi_1 [rad/s] : Inport  Port=4
  Constant3 : Constant  Value=Parameter.Turbine.R_IPC
  InverseColemanTransformation : MATLAB Function  TreatAsAtomicUnit=on
  Product : Product
  Product1 : Product
  v_1 [m/s] : Outport  VectorParamsAs1DForOutWhenUnconnected=off
  v_2 [m/s] : Outport  Port=2  VectorParamsAs1DForOutWhenUnconnected=off
  v_3 [m/s] : Outport  Port=3  VectorParamsAs1DForOutWhenUnconnected=off
  wires:
  Constant3/1 -> Product/2, Product1/1
  v_0 [m/s]/1 -> InverseColemanTransformation/1(x_0)
  delta_H [1/s]/1 -> Product1/2
  InverseColemanTransformation/1(x_1) -> v_1 [m/s]/1  "v_1"
  InverseColemanTransformation/2(x_2) -> v_2 [m/s]/1  "v_2"
  InverseColemanTransformation/3(x_3) -> v_3 [m/s]/1  "v_3"
  Product1/1 -> InverseColemanTransformation/3(x_H)
  Product/1 -> InverseColemanTransformation/2(x_V)
  delta_V [1/s]/1 -> Product/1
  psi_1 [rad/s]/1 -> InverseColemanTransformation/4(psi_1)

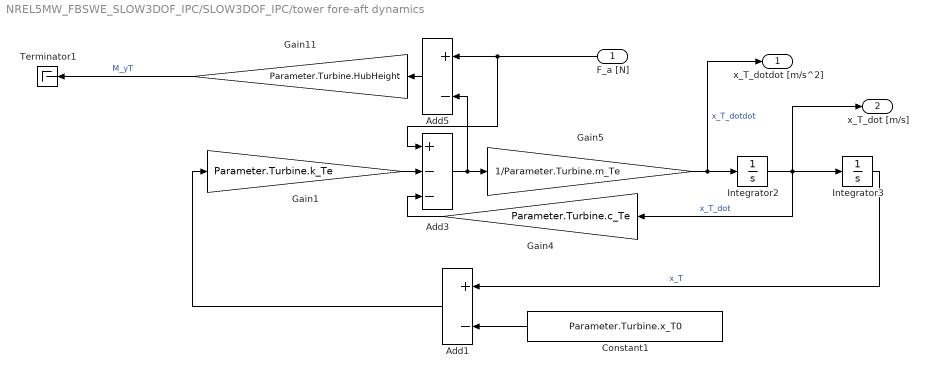
== system NREL5MW_FBSWE_SLOW3DOF_IPC/SLOW3DOF_IPC/tower fore-aft dynamics ==
  F_a [N] : Inport
  Add1 : Sum  Inputs=+-
  Add3 : Sum  Inputs=+--
  Add5 : Sum  Inputs=+-
  Constant1 : Constant  Value=Parameter.Turbine.x_T0
  Gain1 : Gain  Gain=Parameter.Turbine.k_Te  SaturateOnIntegerOverflow=on  OutDataTypeStr=Inherit: Same as input  ParamDataTypeStr=Inherit: Same as input
  Gain11 : Gain  Gain=Parameter.Turbine.HubHeight  SaturateOnIntegerOverflow=on  OutDataTypeStr=Inherit: Same as input  ParamDataTypeStr=Inherit: Same as input
  Gain4 : Gain  Gain=Parameter.Turbine.c_Te  SaturateOnIntegerOverflow=on  OutDataTypeStr=Inherit: Same as input  ParamDataTypeStr=Inherit: Same as input
  Gain5 : Gain  Gain=1/Parameter.Turbine.m_Te  SaturateOnIntegerOverflow=on  OutDataTypeStr=Inherit: Same as input  ParamDataTypeStr=Inherit: Same as input
  Integrator2 : Integrator
  Integrator3 : Integrator  InitialCondition=Parameter.IC.x_T
  Terminator1 : Terminator
  x_T_dotdot [m/s^2] : Outport  VectorParamsAs1DForOutWhenUnconnected=off
  x_T_dot [m/s] : Outport  Port=2  VectorParamsAs1DForOutWhenUnconnected=off
  wires:
  Constant1/1 -> Add1/2
  Add1/1 -> Gain1/1
  Add3/1 -> Gain5/1, Add5/2
  Integrator2/1 -> x_T_dot [m/s]/1, Gain4/1, Integrator3/1  "x_T_dot"
  Integrator3/1 -> Add1/1  "x_T"
  Gain4/1 -> Add3/3
  Gain1/1 -> Add3/2
  Gain5/1 -> x_T_dotdot [m/s^2]/1, Integrator2/1  "x_T_dotdot"
  Add5/1 -> Gain11/1
  Gain11/1 -> Terminator1/1  "M_yT"
  F_a [N]/1 -> Add5/1, Add3/1

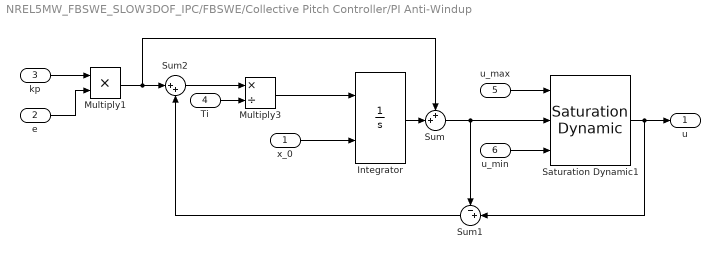
== system NREL5MW_FBSWE_SLOW3DOF_IPC/FBSWE/Collective Pitch Controller/PI Anti-Windup ==
  x_0 : Inport
  e : Inport  Port=2
  kp : Inport  Port=3
  Ti : Inport  Port=4
  u_max : Inport  Port=5
  u_min : Inport  Port=6
  Integrator : Integrator  InitialConditionSource=external
  Multiply1 : Product  Inputs=**
  Multiply3 : Product  Inputs=*/
  Saturation Dynamic1 : simulink/Discontinuities/Saturation Dynamic  OutMin=[]  OutMax=[]  OutDataTypeStr=Inherit: Same as second input  OutDataType=fixdt(1, 16)  OutScaling=2^-10  DoSatur=off
  Sum : Sum  Inputs=++|
  Sum1 : Sum  Inputs=-+|
  Sum2 : Sum  Inputs=|++
  u : Outport  VectorParamsAs1DForOutWhenUnconnected=off
  wires:
  Saturation Dynamic1/1 -> u/1, Sum1/2
  Integrator/1 -> Sum/2
  kp/1 -> Multiply1/1
  e/1 -> Multiply1/2
  Ti/1 -> Multiply3/2
  Sum1/1 -> Sum2/2
  Multiply1/1 -> Sum/1, Sum2/1
  Sum2/1 -> Multiply3/1
  x_0/1 -> Integrator/2
  Multiply3/1 -> Integrator/1
  u_min/1 -> Saturation Dynamic1/3
  Sum/1 -> Saturation Dynamic1/2, Sum1/1
  u_max/1 -> Saturation Dynamic1/1

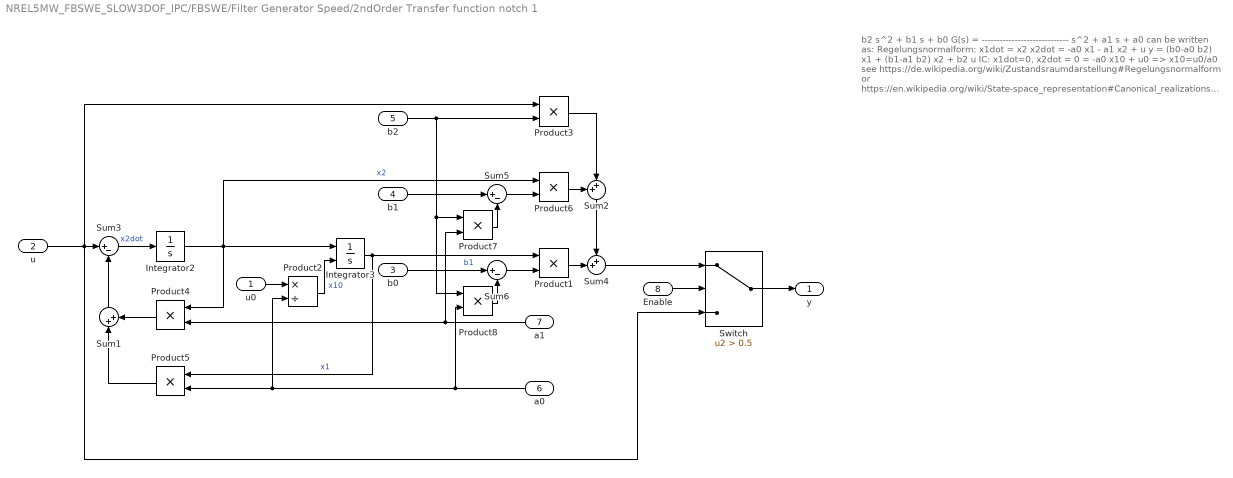
== system NREL5MW_FBSWE_SLOW3DOF_IPC/FBSWE/Filter Generator Speed/2ndOrder Transfer function notch 1 ==
  note: b2 s^2 + b1 s + b0
      | G(s) = -----------------------------
      | s^2 + a1 s + a0
      |
      | can be written as:
      |
      | Regelungsnormalform:
      | x1dot = x2
      | x2dot = -a0 x1 - a1 x2 + u
      | y = (b0-a0 b2) x1 + (b1-a1 b2) x2 + b2 u
      |
      | IC: x1dot=0, x2dot = 0 = -a0 x10 + u0 => x10=u0/a0
      |
      | see https://de.wikipedia.org/wiki/Zustandsraumdarstellung#Regelungsnormalform
      | or
      | https://en.wikipedia.org/wiki/State-space_representation#Canonical_realizations
      |
      | Advantage:
      | - IC can be set
      | - coefficients can be changed online
  u0 : Inport
  u : Inport  Port=2
  b0 : Inport  Port=3
  b1 : Inport  Port=4
  b2 : Inport  Port=5
  a0 : Inport  Port=6
  a1 : Inport  Port=7
  Enable : Inport  Port=8
  Integrator2 : Integrator
  Integrator3 : Integrator  InitialConditionSource=external
  Product{1,3..8} (7 alike) : Product  RndMeth=Zero
  Product2 : Product  Inputs=*/  RndMeth=Zero
  Sum1 : Sum  Inputs=|++
  Sum2 : Sum  Inputs=++|
  Sum3 : Sum  Inputs=|+-
  Sum4 : Sum  Inputs=++|
  Sum5 : Sum  Inputs=|+-
  Sum6 : Sum  Inputs=|+-
  Switch : Switch  Criteria=u2 > Threshold  Threshold=0.5
  y : Outport
  wires:
  Switch/1 -> y/1
  Enable/1 -> Switch/2
  Integrator2/1 -> Integrator3/1, Product6/1, Product4/1  "x2"
  Integrator3/1 -> Product1/1, Product5/1  "x1"
  Sum3/1 -> Integrator2/1  "x2dot"
  u/1 -> Product3/1, Sum3/1, Switch/3
  Sum4/1 -> Switch/1
  Product1/1 -> Sum4/2
  Product6/1 -> Sum2/1
  Sum2/1 -> Sum4/1
  Sum1/1 -> Sum3/2
  Product4/1 -> Sum1/2
  Product5/1 -> Sum1/1
  a0/1 -> Product8/2, Product2/2, Product5/2
  a1/1 -> Product7/2, Product4/2
  b2/1 -> Product8/1, Product7/1, Product3/2
  Product3/1 -> Sum2/2
  Sum5/1 -> Product6/2
  b1/1 -> Sum5/1
  Product7/1 -> Sum5/2
  Sum6/1 -> Product1/2
  b0/1 -> Sum6/1  "b1"
  Product8/1 -> Sum6/2
  Product2/1 -> Integrator3/2  "x10"
  u0/1 -> Product2/1

== system NREL5MW_FBSWE_SLOW3DOF_IPC/FBSWE/Filter Generator Speed/LowPass ==
  u0 : Inport
  u : Inport  Port=2
  f_cutoff : Inport  Port=3
  Enable : Inport  Port=4
  Add3 : Sum  Inputs=-+
  Integrator : Integrator  InitialConditionSource=external
  Product : Product  Inputs=3  RndMeth=Zero
  Switch : Switch  Criteria=u2 > Threshold  Threshold=0.5
  hz to rad : Constant  Value=2*pi
  y : Outport  VectorParamsAs1DForOutWhenUnconnected=off
  wires:
  u0/1 -> Integrator/2
  Switch/1 -> y/1
  Enable/1 -> Switch/2
  u/1 -> Add3/2, Switch/3
  Integrator/1 -> Switch/1, Add3/1
  Product/1 -> Integrator/1
  Add3/1 -> Product/3
  f_cutoff/1 -> Product/2
  hz to rad/1 -> Product/1

== system NREL5MW_FBSWE_SLOW3DOF_IPC/FBSWE/Filter Generator Speed/LowPassDynamicNotchFilter ==
  u0 : Inport
  u : Inport  Port=2
  f_cutoff : Inport  Port=3
  Enable : Inport  Port=4
  Add3 : Sum  Inputs=-+
  Integrator : Integrator  InitialConditionSource=external
  Product : Product  Inputs=3  RndMeth=Zero
  Switch : Switch  Criteria=u2 > Threshold  Threshold=0.5
  hz to rad : Constant  Value=2*pi
  y : Outport  VectorParamsAs1DForOutWhenUnconnected=off
  wires:
  hz to rad/1 -> Product/1
  f_cutoff/1 -> Product/2
  Add3/1 -> Product/3
  Product/1 -> Integrator/1
  Integrator/1 -> Add3/1, Switch/1
  u/1 -> Switch/3, Add3/2
  Enable/1 -> Switch/2
  Switch/1 -> y/1
  u0/1 -> Integrator/2

== system NREL5MW_FBSWE_SLOW3DOF_IPC/FBSWE/Filter Transition/LowPassOrder1 ==
  u0 : Inport
  u : Inport  Port=2
  f_cutoff : Inport  Port=3
  Add3 : Sum  Inputs=-+
  Integrator : Integrator  InitialConditionSource=external
  Product : Product  Inputs=3  RndMeth=Zero
  hz to rad : Constant  Value=2*pi
  y : Outport  VectorParamsAs1DForOutWhenUnconnected=off
  wires:
  u0/1 -> Integrator/2
  Integrator/1 -> y/1, Add3/1
  u/1 -> Add3/2
  Product/1 -> Integrator/1
  Add3/1 -> Product/3
  f_cutoff/1 -> Product/2
  hz to rad/1 -> Product/1

== system NREL5MW_FBSWE_SLOW3DOF_IPC/FBSWE/Torque Controller/LimitsAndReferenceValueTC ==
  Omega_g [rad/s] : Inport
  Delta_Omega_g [rad/s] : Inport  Port=2
  Constant1 : Constant  Value=Parameter.VSC.Omega_g_1d5
  Constant2 : Constant  Value=Parameter.VSC.M_g_rated
  Constant3 : Constant  Value=Parameter.VSC.k
  Constant5 : Constant  Value=Parameter.CPC.Omega_g_rated
  Constant6 : Constant  Value=Parameter.VSC.M_g_max
  LimitsAndReferenceValueTC : MATLAB Function  TreatAsAtomicUnit=on
  Omega_g_ref [rad/s] : Outport  VectorParamsAs1DForOutWhenUnconnected=off
  M_g_ub [Nm] : Outport  Port=2  VectorParamsAs1DForOutWhenUnconnected=off
  M_g_lb [Nm] : Outport  Port=3  VectorParamsAs1DForOutWhenUnconnected=off
  wires:
  LimitsAndReferenceValueTC/2(M_g_ub) -> M_g_ub [Nm]/1  "M_g_ub"
  Omega_g [rad/s]/1 -> LimitsAndReferenceValueTC/1(Omega_g)
  Constant1/1 -> LimitsAndReferenceValueTC/3(Omega_g_1d5)
  Constant3/1 -> LimitsAndReferenceValueTC/4(k)
  Constant2/1 -> LimitsAndReferenceValueTC/6(M_g_rated)
  Constant5/1 -> LimitsAndReferenceValueTC/5(Omega_g_rated)
  LimitsAndReferenceValueTC/1(Omega_g_ref) -> Omega_g_ref [rad/s]/1  "Omega_g_ref"
  LimitsAndReferenceValueTC/3(M_g_lb) -> M_g_lb [Nm]/1  "M_g_lb"
  Constant6/1 -> LimitsAndReferenceValueTC/7(M_g_max)
  Delta_Omega_g [rad/s]/1 -> LimitsAndReferenceValueTC/2(Delta_Omega_g)

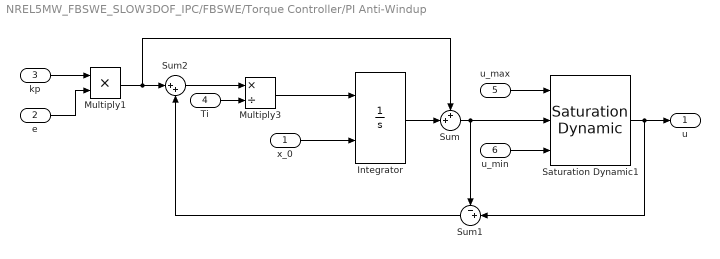
== system NREL5MW_FBSWE_SLOW3DOF_IPC/FBSWE/Torque Controller/PI Anti-Windup ==
  x_0 : Inport
  e : Inport  Port=2
  kp : Inport  Port=3
  Ti : Inport  Port=4
  u_max : Inport  Port=5
  u_min : Inport  Port=6
  Integrator : Integrator  InitialConditionSource=external
  Multiply1 : Product  Inputs=**
  Multiply3 : Product  Inputs=*/
  Saturation Dynamic1 : simulink/Discontinuities/Saturation Dynamic  OutMin=[]  OutMax=[]  OutDataTypeStr=Inherit: Same as second input  OutDataType=fixdt(1, 16)  OutScaling=2^-10  DoSatur=off
  Sum : Sum  Inputs=++|
  Sum1 : Sum  Inputs=-+|
  Sum2 : Sum  Inputs=|++
  u : Outport  VectorParamsAs1DForOutWhenUnconnected=off
  wires:
  Saturation Dynamic1/1 -> u/1, Sum1/2
  Integrator/1 -> Sum/2
  kp/1 -> Multiply1/1
  e/1 -> Multiply1/2
  Ti/1 -> Multiply3/2
  Sum1/1 -> Sum2/2
  Multiply1/1 -> Sum/1, Sum2/1
  Sum2/1 -> Multiply3/1
  x_0/1 -> Integrator/2
  Multiply3/1 -> Integrator/1
  u_min/1 -> Saturation Dynamic1/3
  Sum/1 -> Saturation Dynamic1/2, Sum1/1
  u_max/1 -> Saturation Dynamic1/1

== system NREL5MW_FBSWE_SLOW3DOF_IPC/SLOW3DOF_IPC/aerodynamics/aerodynamics blade 1 ==
  Omega [rad/s] : Inport
  v_i [m/s] : Inport  Port=2
  x_T_dot [m/s] : Inport  Port=3
  theta_i [rad] : Inport  Port=4
  Aerodynamic Thrust : Subsystem
  Aerodynamic Torque : Subsystem
  Gain : Gain  Gain=1/3
  Gain1 : Gain  Gain=1/3
  Tip Speed Ratio : Subsystem
  relative Wind Speed : Subsystem
  M_a_i [Nm] : Outport  VectorParamsAs1DForOutWhenUnconnected=off
  F_a_i [N] : Outport  Port=2  VectorParamsAs1DForOutWhenUnconnected=off
  wires:
  theta_i [rad]/1 -> Aerodynamic Thrust/1(theta [rad]), Aerodynamic Torque/1(theta [rad])
  Aerodynamic Torque/1(M_a [Nm]) -> Gain1/1
  Aerodynamic Thrust/1(F_a [N]) -> Gain/1
  x_T_dot [m/s]/1 -> relative Wind Speed/2(x_T_dot [m/s])
  v_i [m/s]/1 -> relative Wind Speed/1(v_0 [m/s])
  Omega [rad/s]/1 -> Tip Speed Ratio/1(Omega [rad/s])
  relative Wind Speed/1(v_rel [m/s]) -> Tip Speed Ratio/2(v_rel [m/s]), Aerodynamic Torque/3(v_rel [m/s]), Aerodynamic Thrust/3(v_rel [m/s])
  Tip Speed Ratio/1(lambda [-]) -> Aerodynamic Thrust/2(lambda [-]), Aerodynamic Torque/2(lambda [-])  "lambda"
  Gain/1 -> F_a_i [N]/1
  Gain1/1 -> M_a_i [Nm]/1

== system NREL5MW_FBSWE_SLOW3DOF_IPC/SLOW3DOF_IPC/aerodynamics/aerodynamics blade 2 ==
  Omega [rad/s] : Inport
  v_i [m/s] : Inport  Port=2
  x_T_dot [m/s] : Inport  Port=3
  theta_i [rad] : Inport  Port=4
  Aerodynamic Thrust : Subsystem
  Aerodynamic Torque : Subsystem
  Gain : Gain  Gain=1/3
  Gain1 : Gain  Gain=1/3
  Tip Speed Ratio : Subsystem
  relative Wind Speed : Subsystem
  M_a_i [Nm] : Outport  VectorParamsAs1DForOutWhenUnconnected=off
  F_a_i [N] : Outport  Port=2  VectorParamsAs1DForOutWhenUnconnected=off
  wires:
  Gain1/1 -> M_a_i [Nm]/1
  Gain/1 -> F_a_i [N]/1
  Tip Speed Ratio/1(lambda [-]) -> Aerodynamic Torque/2(lambda [-]), Aerodynamic Thrust/2(lambda [-])  "lambda"
  relative Wind Speed/1(v_rel [m/s]) -> Aerodynamic Thrust/3(v_rel [m/s]), Aerodynamic Torque/3(v_rel [m/s]), Tip Speed Ratio/2(v_rel [m/s])
  Omega [rad/s]/1 -> Tip Speed Ratio/1(Omega [rad/s])
  v_i [m/s]/1 -> relative Wind Speed/1(v_0 [m/s])
  x_T_dot [m/s]/1 -> relative Wind Speed/2(x_T_dot [m/s])
  Aerodynamic Thrust/1(F_a [N]) -> Gain/1
  Aerodynamic Torque/1(M_a [Nm]) -> Gain1/1
  theta_i [rad]/1 -> Aerodynamic Torque/1(theta [rad]), Aerodynamic Thrust/1(theta [rad])

== system NREL5MW_FBSWE_SLOW3DOF_IPC/SLOW3DOF_IPC/aerodynamics/aerodynamics blade 3 ==
  Omega [rad/s] : Inport
  v_i [m/s] : Inport  Port=2
  x_T_dot [m/s] : Inport  Port=3
  theta_i [rad] : Inport  Port=4
  Aerodynamic Thrust : Subsystem
  Aerodynamic Torque : Subsystem
  Gain : Gain  Gain=1/3
  Gain1 : Gain  Gain=1/3
  Tip Speed Ratio : Subsystem
  relative Wind Speed : Subsystem
  M_a_i [Nm] : Outport  VectorParamsAs1DForOutWhenUnconnected=off
  F_a_i [N] : Outport  Port=2  VectorParamsAs1DForOutWhenUnconnected=off
  wires:
  theta_i [rad]/1 -> Aerodynamic Thrust/1(theta [rad]), Aerodynamic Torque/1(theta [rad])
  Aerodynamic Torque/1(M_a [Nm]) -> Gain1/1
  Aerodynamic Thrust/1(F_a [N]) -> Gain/1
  x_T_dot [m/s]/1 -> relative Wind Speed/2(x_T_dot [m/s])
  v_i [m/s]/1 -> relative Wind Speed/1(v_0 [m/s])
  Omega [rad/s]/1 -> Tip Speed Ratio/1(Omega [rad/s])
  relative Wind Speed/1(v_rel [m/s]) -> Tip Speed Ratio/2(v_rel [m/s]), Aerodynamic Torque/3(v_rel [m/s]), Aerodynamic Thrust/3(v_rel [m/s])
  Tip Speed Ratio/1(lambda [-]) -> Aerodynamic Thrust/2(lambda [-]), Aerodynamic Torque/2(lambda [-])  "lambda"
  Gain/1 -> F_a_i [N]/1
  Gain1/1 -> M_a_i [Nm]/1

== system NREL5MW_FBSWE_SLOW3DOF_IPC/SLOW3DOF_IPC/pitch actuators/Pitch Actuator 1 ==
  u : Inport
  y0 : Inport  Port=2
  Add3 : Sum  Inputs=+--
  Gain1 : Gain  Gain=omega*omega  SaturateOnIntegerOverflow=on  OutDataTypeStr=Inherit: Same as input  ParamDataTypeStr=Inherit: Same as input
  Gain2 : Gain  Gain=omega*omega  SaturateOnIntegerOverflow=on  OutDataTypeStr=Inherit: Same as input  ParamDataTypeStr=Inherit: Same as input
  Gain3 : Gain  Gain=2*xi*omega  SaturateOnIntegerOverflow=on  OutDataTypeStr=Inherit: Same as input  ParamDataTypeStr=Inherit: Same as input
  Integrator1 : Integrator  LimitOutput=on  UpperSaturationLimit=x1_max  LowerSaturationLimit=x1_min
  Integrator2 : Integrator  InitialConditionSource=external  InitialCondition=x2_t0  UpperSaturationLimit=x2_max  LowerSaturationLimit=x2_min
  y : Outport  VectorParamsAs1DForOutWhenUnconnected=off
  x1 : Outport  Port=2  VectorParamsAs1DForOutWhenUnconnected=off
  wires:
  Gain3/1 -> Add3/3
  u/1 -> Gain1/1
  Add3/1 -> Integrator1/1
  Gain1/1 -> Add3/1
  Gain2/1 -> Add3/2
  Integrator1/1 -> x1/1, Gain3/1, Integrator2/1  "x1"
  y0/1 -> Integrator2/2
  Integrator2/1 -> Gain2/1, y/1

== system NREL5MW_FBSWE_SLOW3DOF_IPC/SLOW3DOF_IPC/pitch actuators/Pitch Actuator 2 ==
  u : Inport
  y0 : Inport  Port=2
  Add3 : Sum  Inputs=+--
  Gain1 : Gain  Gain=omega*omega  SaturateOnIntegerOverflow=on  OutDataTypeStr=Inherit: Same as input  ParamDataTypeStr=Inherit: Same as input
  Gain2 : Gain  Gain=omega*omega  SaturateOnIntegerOverflow=on  OutDataTypeStr=Inherit: Same as input  ParamDataTypeStr=Inherit: Same as input
  Gain3 : Gain  Gain=2*xi*omega  SaturateOnIntegerOverflow=on  OutDataTypeStr=Inherit: Same as input  ParamDataTypeStr=Inherit: Same as input
  Integrator1 : Integrator  LimitOutput=on  UpperSaturationLimit=x1_max  LowerSaturationLimit=x1_min
  Integrator2 : Integrator  InitialConditionSource=external  InitialCondition=x2_t0  UpperSaturationLimit=x2_max  LowerSaturationLimit=x2_min
  y : Outport  VectorParamsAs1DForOutWhenUnconnected=off
  x1 : Outport  Port=2  VectorParamsAs1DForOutWhenUnconnected=off
  wires:
  Integrator2/1 -> y/1, Gain2/1
  y0/1 -> Integrator2/2
  Integrator1/1 -> Integrator2/1, Gain3/1, x1/1  "x1"
  Gain2/1 -> Add3/2
  Gain1/1 -> Add3/1
  Add3/1 -> Integrator1/1
  u/1 -> Gain1/1
  Gain3/1 -> Add3/3

== system NREL5MW_FBSWE_SLOW3DOF_IPC/SLOW3DOF_IPC/pitch actuators/Pitch Actuator 3 ==
  u : Inport
  y0 : Inport  Port=2
  Add3 : Sum  Inputs=+--
  Gain1 : Gain  Gain=omega*omega  SaturateOnIntegerOverflow=on  OutDataTypeStr=Inherit: Same as input  ParamDataTypeStr=Inherit: Same as input
  Gain2 : Gain  Gain=omega*omega  SaturateOnIntegerOverflow=on  OutDataTypeStr=Inherit: Same as input  ParamDataTypeStr=Inherit: Same as input
  Gain3 : Gain  Gain=2*xi*omega  SaturateOnIntegerOverflow=on  OutDataTypeStr=Inherit: Same as input  ParamDataTypeStr=Inherit: Same as input
  Integrator1 : Integrator  LimitOutput=on  UpperSaturationLimit=x1_max  LowerSaturationLimit=x1_min
  Integrator2 : Integrator  InitialConditionSource=external  InitialCondition=x2_t0  UpperSaturationLimit=x2_max  LowerSaturationLimit=x2_min
  y : Outport  VectorParamsAs1DForOutWhenUnconnected=off
  x1 : Outport  Port=2  VectorParamsAs1DForOutWhenUnconnected=off
  wires:
  Gain3/1 -> Add3/3
  u/1 -> Gain1/1
  Add3/1 -> Integrator1/1
  Gain1/1 -> Add3/1
  Gain2/1 -> Add3/2
  Integrator1/1 -> x1/1, Gain3/1, Integrator2/1  "x1"
  y0/1 -> Integrator2/2
  Integrator2/1 -> Gain2/1, y/1

== system NREL5MW_FBSWE_SLOW3DOF_IPC/SLOW3DOF_IPC/aerodynamics/aerodynamics blade 1/Aerodynamic Thrust ==
  theta [rad] : Inport
  lambda [-] : Inport  Port=2
  v_rel [m/s] : Inport  Port=3
  Fcn1 : Fcn  Expr=1/2*Parameter.General.rho*pi*Parameter.Turbine.R^2*u(1)
  Product1 : Product  Inputs=3  RndMeth=Zero
  effective force coefficient : Lookup2D  RowIndex=Parameter.Turbine.SS.lambda  ColumnIndex=Parameter.Turbine.SS.theta  Table=Parameter.Turbine.SS.c_T
  F_a [N] : Outport  VectorParamsAs1DForOutWhenUnconnected=off
  wires:
  v_rel [m/s]/1 -> Product1/2, Product1/1
  theta [rad]/1 -> effective force coefficient/2
  lambda [-]/1 -> effective force coefficient/1
  Fcn1/1 -> Product1/3
  Product1/1 -> F_a [N]/1  "F_a"
  effective force coefficient/1 -> Fcn1/1  "c_T"

== system NREL5MW_FBSWE_SLOW3DOF_IPC/SLOW3DOF_IPC/aerodynamics/aerodynamics blade 1/Aerodynamic Torque ==
  theta [rad] : Inport
  lambda [-] : Inport  Port=2
  v_rel [m/s] : Inport  Port=3
  Fcn1 : Fcn  Expr=1/2*Parameter.General.rho*pi*Parameter.Turbine.R^3*u(1)
  Product1 : Product  Inputs=3  RndMeth=Zero
  Product2 : Product  Inputs=/*  RndMeth=Zero
  effective power coefficient : Lookup2D  RowIndex=Parameter.Turbine.SS.lambda  ColumnIndex=Parameter.Turbine.SS.theta  Table=Parameter.Turbine.SS.c_P
  M_a [Nm] : Outport  VectorParamsAs1DForOutWhenUnconnected=off
  wires:
  Product1/1 -> M_a [Nm]/1  "M_a"
  Fcn1/1 -> Product1/3
  lambda [-]/1 -> effective power coefficient/1, Product2/1
  theta [rad]/1 -> effective power coefficient/2
  v_rel [m/s]/1 -> Product1/1, Product1/2
  effective power coefficient/1 -> Product2/2  "c_P"
  Product2/1 -> Fcn1/1

== system NREL5MW_FBSWE_SLOW3DOF_IPC/SLOW3DOF_IPC/aerodynamics/aerodynamics blade 1/Tip Speed Ratio ==
  Omega [rad/s] : Inport
  v_rel [m/s] : Inport  Port=2
  Gain6 : Gain  Gain=Parameter.Turbine.R  SaturateOnIntegerOverflow=on  OutDataTypeStr=Inherit: Same as input  ParamDataTypeStr=Inherit: Same as input
  Product3 : Product  Inputs=*/  RndMeth=Zero
  lambda [-] : Outport  VectorParamsAs1DForOutWhenUnconnected=off
  wires:
  Product3/1 -> Gain6/1
  Omega [rad/s]/1 -> Product3/1
  v_rel [m/s]/1 -> Product3/2
  Gain6/1 -> lambda [-]/1  "lambda"

== system NREL5MW_FBSWE_SLOW3DOF_IPC/SLOW3DOF_IPC/aerodynamics/aerodynamics blade 1/relative Wind Speed ==
  v_0 [m/s] : Inport
  x_T_dot [m/s] : Inport  Port=2
  Add2 : Sum  Inputs=-+
  v_rel [m/s] : Outport  VectorParamsAs1DForOutWhenUnconnected=off
  wires:
  Add2/1 -> v_rel [m/s]/1  "v_rel"
  x_T_dot [m/s]/1 -> Add2/1
  v_0 [m/s]/1 -> Add2/2

== system NREL5MW_FBSWE_SLOW3DOF_IPC/SLOW3DOF_IPC/aerodynamics/aerodynamics blade 2/Aerodynamic Thrust ==
  theta [rad] : Inport
  lambda [-] : Inport  Port=2
  v_rel [m/s] : Inport  Port=3
  Fcn1 : Fcn  Expr=1/2*Parameter.General.rho*pi*Parameter.Turbine.R^2*u(1)
  Product1 : Product  Inputs=3  RndMeth=Zero
  effective force coefficient : Lookup2D  RowIndex=Parameter.Turbine.SS.lambda  ColumnIndex=Parameter.Turbine.SS.theta  Table=Parameter.Turbine.SS.c_T
  F_a [N] : Outport  VectorParamsAs1DForOutWhenUnconnected=off
  wires:
  effective force coefficient/1 -> Fcn1/1  "c_T"
  Product1/1 -> F_a [N]/1  "F_a"
  Fcn1/1 -> Product1/3
  lambda [-]/1 -> effective force coefficient/1
  theta [rad]/1 -> effective force coefficient/2
  v_rel [m/s]/1 -> Product1/1, Product1/2

== system NREL5MW_FBSWE_SLOW3DOF_IPC/SLOW3DOF_IPC/aerodynamics/aerodynamics blade 2/Aerodynamic Torque ==
  theta [rad] : Inport
  lambda [-] : Inport  Port=2
  v_rel [m/s] : Inport  Port=3
  Fcn1 : Fcn  Expr=1/2*Parameter.General.rho*pi*Parameter.Turbine.R^3*u(1)
  Product1 : Product  Inputs=3  RndMeth=Zero
  Product2 : Product  Inputs=/*  RndMeth=Zero
  effective power coefficient : Lookup2D  RowIndex=Parameter.Turbine.SS.lambda  ColumnIndex=Parameter.Turbine.SS.theta  Table=Parameter.Turbine.SS.c_P
  M_a [Nm] : Outport  VectorParamsAs1DForOutWhenUnconnected=off
  wires:
  Product2/1 -> Fcn1/1
  effective power coefficient/1 -> Product2/2  "c_P"
  v_rel [m/s]/1 -> Product1/2, Product1/1
  theta [rad]/1 -> effective power coefficient/2
  lambda [-]/1 -> Product2/1, effective power coefficient/1
  Fcn1/1 -> Product1/3
  Product1/1 -> M_a [Nm]/1  "M_a"

== system NREL5MW_FBSWE_SLOW3DOF_IPC/SLOW3DOF_IPC/aerodynamics/aerodynamics blade 2/Tip Speed Ratio ==
  Omega [rad/s] : Inport
  v_rel [m/s] : Inport  Port=2
  Gain6 : Gain  Gain=Parameter.Turbine.R  SaturateOnIntegerOverflow=on  OutDataTypeStr=Inherit: Same as input  ParamDataTypeStr=Inherit: Same as input
  Product3 : Product  Inputs=*/  RndMeth=Zero
  lambda [-] : Outport  VectorParamsAs1DForOutWhenUnconnected=off
  wires:
  Gain6/1 -> lambda [-]/1  "lambda"
  v_rel [m/s]/1 -> Product3/2
  Omega [rad/s]/1 -> Product3/1
  Product3/1 -> Gain6/1

== system NREL5MW_FBSWE_SLOW3DOF_IPC/SLOW3DOF_IPC/aerodynamics/aerodynamics blade 2/relative Wind Speed ==
  v_0 [m/s] : Inport
  x_T_dot [m/s] : Inport  Port=2
  Add2 : Sum  Inputs=-+
  v_rel [m/s] : Outport  VectorParamsAs1DForOutWhenUnconnected=off
  wires:
  v_0 [m/s]/1 -> Add2/2
  x_T_dot [m/s]/1 -> Add2/1
  Add2/1 -> v_rel [m/s]/1  "v_rel"

== system NREL5MW_FBSWE_SLOW3DOF_IPC/SLOW3DOF_IPC/aerodynamics/aerodynamics blade 3/Aerodynamic Thrust ==
  theta [rad] : Inport
  lambda [-] : Inport  Port=2
  v_rel [m/s] : Inport  Port=3
  Fcn1 : Fcn  Expr=1/2*Parameter.General.rho*pi*Parameter.Turbine.R^2*u(1)
  Product1 : Product  Inputs=3  RndMeth=Zero
  effective force coefficient : Lookup2D  RowIndex=Parameter.Turbine.SS.lambda  ColumnIndex=Parameter.Turbine.SS.theta  Table=Parameter.Turbine.SS.c_T
  F_a [N] : Outport  VectorParamsAs1DForOutWhenUnconnected=off
  wires:
  v_rel [m/s]/1 -> Product1/2, Product1/1
  theta [rad]/1 -> effective force coefficient/2
  lambda [-]/1 -> effective force coefficient/1
  Fcn1/1 -> Product1/3
  Product1/1 -> F_a [N]/1  "F_a"
  effective force coefficient/1 -> Fcn1/1  "c_T"

== system NREL5MW_FBSWE_SLOW3DOF_IPC/SLOW3DOF_IPC/aerodynamics/aerodynamics blade 3/Aerodynamic Torque ==
  theta [rad] : Inport
  lambda [-] : Inport  Port=2
  v_rel [m/s] : Inport  Port=3
  Fcn1 : Fcn  Expr=1/2*Parameter.General.rho*pi*Parameter.Turbine.R^3*u(1)
  Product1 : Product  Inputs=3  RndMeth=Zero
  Product2 : Product  Inputs=/*  RndMeth=Zero
  effective power coefficient : Lookup2D  RowIndex=Parameter.Turbine.SS.lambda  ColumnIndex=Parameter.Turbine.SS.theta  Table=Parameter.Turbine.SS.c_P
  M_a [Nm] : Outport  VectorParamsAs1DForOutWhenUnconnected=off
  wires:
  Product1/1 -> M_a [Nm]/1  "M_a"
  Fcn1/1 -> Product1/3
  lambda [-]/1 -> effective power coefficient/1, Product2/1
  theta [rad]/1 -> effective power coefficient/2
  v_rel [m/s]/1 -> Product1/1, Product1/2
  effective power coefficient/1 -> Product2/2  "c_P"
  Product2/1 -> Fcn1/1

== system NREL5MW_FBSWE_SLOW3DOF_IPC/SLOW3DOF_IPC/aerodynamics/aerodynamics blade 3/Tip Speed Ratio ==
  Omega [rad/s] : Inport
  v_rel [m/s] : Inport  Port=2
  Gain6 : Gain  Gain=Parameter.Turbine.R  SaturateOnIntegerOverflow=on  OutDataTypeStr=Inherit: Same as input  ParamDataTypeStr=Inherit: Same as input
  Product3 : Product  Inputs=*/  RndMeth=Zero
  lambda [-] : Outport  VectorParamsAs1DForOutWhenUnconnected=off
  wires:
  Product3/1 -> Gain6/1
  Omega [rad/s]/1 -> Product3/1
  v_rel [m/s]/1 -> Product3/2
  Gain6/1 -> lambda [-]/1  "lambda"

== system NREL5MW_FBSWE_SLOW3DOF_IPC/SLOW3DOF_IPC/aerodynamics/aerodynamics blade 3/relative Wind Speed ==
  v_0 [m/s] : Inport
  x_T_dot [m/s] : Inport  Port=2
  Add2 : Sum  Inputs=-+
  v_rel [m/s] : Outport  VectorParamsAs1DForOutWhenUnconnected=off
  wires:
  Add2/1 -> v_rel [m/s]/1  "v_rel"
  x_T_dot [m/s]/1 -> Add2/1
  v_0 [m/s]/1 -> Add2/2

== matlab function NREL5MW_FBSWE_SLOW3DOF_IPC/FBSWE/Individual Pitch Controllers/InverseColemanTransformation ==
  data: x_1 output; x_2 output; x_3 output; x_0 input; x_V input; x_H input; psi_1 input
function [x_1,x_2,x_3] = InverseColemanTransformation(x_0,x_V,x_H,psi_1)

% inverse Coleman Transformation
x_1 = 0; % Dummy
x_2 = 0; % Dummy
x_3 = 0; % Dummy   

end

== matlab function NREL5MW_FBSWE_SLOW3DOF_IPC/SLOW3DOF_IPC/rotational sampling wind/InverseColemanTransformation ==
  settings: fimath=|
      | fimath(...
      | 'RoundMode', 'floor',...
      | 'OverflowMode', 'wrap',...
      | 'ProductMode', 'KeepLSB', 'ProductWordLength', 32,...
      | 'SumMode', 'KeepLSB', 'SumWordLength', 32,...
      | 'CastBeforeSum', false)
  data: x_1 output; x_2 output; x_3 output; x_0 input; x_V input; x_H input; psi_1 input
function [x_1,x_2,x_3] = InverseColemanTransformation(x_0,x_V,x_H,psi_1)

% the other 2 azimut angles
psi_2 = psi_1 + 2/3*pi;
psi_3 = psi_2 + 2/3*pi;

% inverse Coleman Transformation
x_1 = x_0 + cos(psi_1) * x_V + sin(psi_1) * x_H;
x_2 = x_0 + cos(psi_2) * x_V + sin(psi_2) * x_H;
x_3 = x_0 + cos(psi_3) * x_V + sin(psi_3) * x_H;

end
